simulink model "slx0014"  (Simulink 9.2)
settings: Solver=FixedStepDiscrete  StartTime=0.0  StopTime=Tsim  FixedStep=grampc.param.dt  RelTol=1e-3  EnableMultiTasking=on
undefined symbols (not defined in the file): grampc
settings Model: Creator=kaepernick  LastModifiedBy=sacredsky
settings DataIOCC: SignalLoggingSaveFormat=Dataset
settings OptimizationCC: ExpressionDepthLimit=2147483647
settings DebuggingCC: SolverPrmCheckMsg=warning  FcnCallInpInsideContextMsg=error
settings GRTTargetCC: CombineOutputUpdateFcns=on  GRTInterface=off

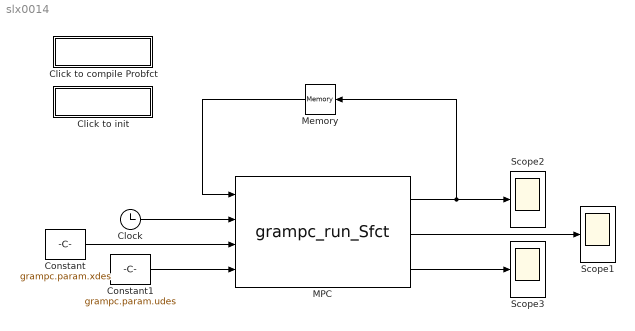
== system slx0014 ==
  Click to compile Probfct : Subsystem
      settings: OpenFcn=|
      | cd(fileparts(which(gcs)))
      |     if exist('make','file') ~= 2
      |       curPath = cd;
      |       cd('..');
      |       addpath(cd);
      |       cd(curPath);
      |     end
      | make probfct_REACTOR_CSTR.c
  Click to init : Subsystem
      settings: OpenFcn=|
      | cd(fileparts(which(gcs)))
      | [grampc,Tsim] = initData;
  Clock : Clock
  Constant : Constant  Value=grampc.param.xdes
  Constant1 : Constant  Value=grampc.param.udes
  MPC : S-Function  FunctionName=grampc_run_Sfct  Parameters=grampc  SFunctionDeploymentMode=off  EnableBusSupport=off
      mask Display:
      | port_label('input',1,'xk')
      | port_label('input',2,'tk')
      | port_label('input',3,'xdes')
      | port_label('input',4,'udes')
      | 
      | port_label('output',1,'xnext')
      | port_label('output',2,'unext')
      | port_label('output',3,'cost')
  Memory : Memory  InitialCondition=grampc.param.xk
  Scope1 : Scope
  Scope2 : Scope
  Scope3 : Scope
  wires:
  MPC/1 -> Memory/1, Scope2/1
  MPC/2 -> Scope1/1
  MPC/3 -> Scope3/1
  Memory/1 -> MPC/1
  Clock/1 -> MPC/2
  Constant1/1 -> MPC/4
  Constant/1 -> MPC/3

== system slx0014/Click to compile Probfct ==

== system slx0014/Click to init ==
